simulink model "simplified_sim_2018"  (R2018b)
settings: Solver=VariableStepAuto  StartTime=0.0  StopTime=10.0  RelTol=1e-3
undefined symbols (not defined in the file or in its folder): sensors
libraries: dspindex x4, Environment_lib x1, Sensors_Lib x1, MEKF_lib x1, satelliteDynamics_lib x1
settings Model: Creator=satcave1  LastModifiedBy=kylle

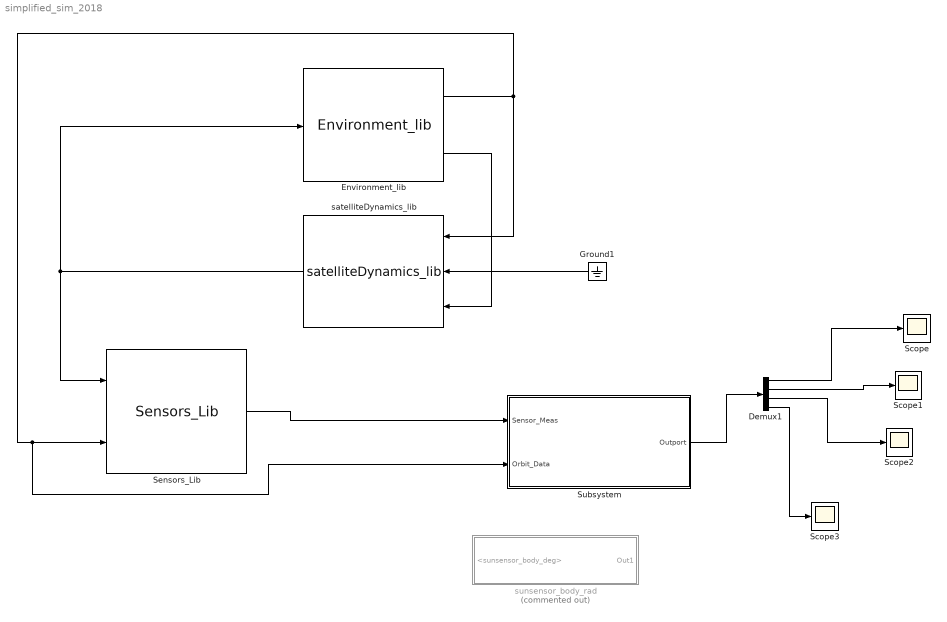
== system simplified_sim_2018 ==
  Demux1 : Demux
  Environment_lib : Environment_lib/Environment_lib  SystemSampleTime=-1
  Ground1 : Ground
  Scope{,1..3} (4 alike) : Scope
  Sensors_Lib : Sensors_Lib/Sensors_Lib  SystemSampleTime=-1
  Subsystem : Subsystem
  satelliteDynamics_lib : satelliteDynamics_lib/satelliteDynamics_lib  SystemSampleTime=-1
  sunsensor_body_rad : Subsystem  Commented=on
  wires:
  satelliteDynamics_lib/1 -> Environment_lib/1, Sensors_Lib/1
  Ground1/1 -> satelliteDynamics_lib/2
  Environment_lib/2 -> satelliteDynamics_lib/3
  Environment_lib/1 -> Subsystem/2(Orbit_Data), Sensors_Lib/2, satelliteDynamics_lib/1
  Sensors_Lib/1 -> Subsystem/1(Sensor_Meas)
  Subsystem/1(Outport) -> Demux1/1
  Demux1/1 -> Scope/1
  Demux1/2 -> Scope1/1
  Demux1/3 -> Scope2/1
  Demux1/4 -> Scope3/1

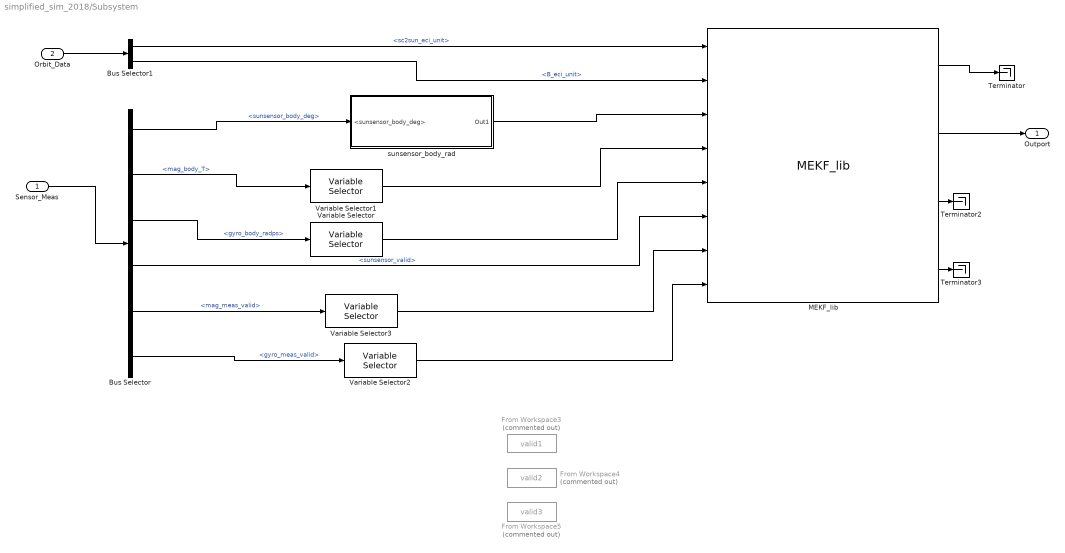
== system simplified_sim_2018/Subsystem ==
  Sensor_Meas : Inport
  Orbit_Data : Inport  Port=2
  Bus Selector : BusSelector  OutputSignals=sunsensor_body_deg,mag_body_T,gyro_body_radps,sunsensor_valid,mag_meas_valid,gyro_meas_valid
  Bus Selector1 : BusSelector  OutputSignals=sc2sun_eci_unit,B_eci_unit
  From Workspace3 : FromWorkspace  Commented=on  VariableName=valid1  SampleTime=sensors.sample_time_s
  From Workspace4 : FromWorkspace  Commented=on  VariableName=valid2  SampleTime=sensors.sample_time_s
  From Workspace5 : FromWorkspace  Commented=on  VariableName=valid3  SampleTime=sensors.sample_time_s
  MEKF_lib : MEKF_lib/MEKF_lib  SystemSampleTime=-1
  Terminator : Terminator
  Terminator2 : Terminator
  Terminator3 : Terminator
  Variable Selector : dspindex/Variable Selector  NumInputs=1  rowsOrCols=Columns  IdxMode=Fixed  Elements=[1]  ZerOneIdxMode=One-based  errmode=Clip Index  FillMode=off  FillValues=0
  Variable Selector1 : dspindex/Variable Selector  NumInputs=1  rowsOrCols=Columns  IdxMode=Fixed  Elements=[1]  ZerOneIdxMode=One-based  errmode=Clip Index  FillMode=off  FillValues=0
  Variable Selector2 : dspindex/Variable Selector  NumInputs=1  rowsOrCols=Rows  IdxMode=Fixed  Elements=[1]  ZerOneIdxMode=One-based  errmode=Clip Index  FillMode=off  FillValues=0
  Variable Selector3 : dspindex/Variable Selector  NumInputs=1  rowsOrCols=Rows  IdxMode=Fixed  Elements=[1]  ZerOneIdxMode=One-based  errmode=Clip Index  FillMode=off  FillValues=0
  sunsensor_body_rad : Subsystem
  Outport : Outport
  wires:
  MEKF_lib/1 -> Terminator/1
  MEKF_lib/2 -> Outport/1
  MEKF_lib/3 -> Terminator2/1
  MEKF_lib/4 -> Terminator3/1
  Sensor_Meas/1 -> Bus Selector/1
  Orbit_Data/1 -> Bus Selector1/1
  Bus Selector1/1 -> MEKF_lib/1  "<sc2sun_eci_unit>"
  Bus Selector1/2 -> MEKF_lib/2  "<B_eci_unit>"
  sunsensor_body_rad/1(Out1) -> MEKF_lib/3
  Bus Selector/1 -> sunsensor_body_rad/1(<sunsensor_body_deg>)  "<sunsensor_body_deg>"
  Bus Selector/3 -> Variable Selector/1  "<gyro_body_radps>"
  Bus Selector/2 -> Variable Selector1/1  "<mag_body_T>"
  Variable Selector1/1 -> MEKF_lib/4
  Variable Selector/1 -> MEKF_lib/5
  Bus Selector/4 -> MEKF_lib/6  "<sunsensor_valid>"
  Bus Selector/6 -> Variable Selector2/1  "<gyro_meas_valid>"
  Variable Selector2/1 -> MEKF_lib/8
  Bus Selector/5 -> Variable Selector3/1  "<mag_meas_valid>"
  Variable Selector3/1 -> MEKF_lib/7

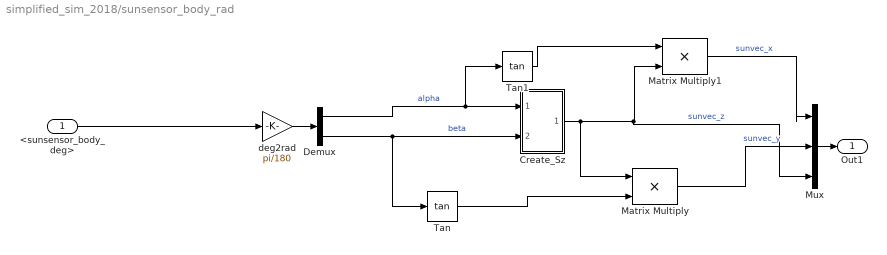
== system simplified_sim_2018/sunsensor_body_rad ==
  <sunsensor_body_deg> : Inport
  Create_Sz : Subsystem
  Demux : Demux  Outputs=2
  Matrix Multiply : Product
  Matrix Multiply1 : Product
  Mux : Mux  Inputs=3
  Tan : Trigonometry  Operator=tan
  Tan1 : Trigonometry  Operator=tan
  deg2rad : Gain  Gain=pi/180
  Out1 : Outport
  wires:
  Tan/1 -> Matrix Multiply/2
  Demux/1 -> Tan1/1, Create_Sz/1(alpha)  "alpha"
  Matrix Multiply/1 -> Mux/2  "sunvec_y"
  Create_Sz/1(Out1) -> Mux/3, Matrix Multiply1/2, Matrix Multiply/1  "sunvec_z"
  Demux/2 -> Tan/1, Create_Sz/2(beta)  "beta"
  Tan1/1 -> Matrix Multiply1/1
  deg2rad/1 -> Demux/1
  Mux/1 -> Out1/1
  Matrix Multiply1/1 -> Mux/1  "sunvec_x"
  <sunsensor_body_deg>/1 -> deg2rad/1

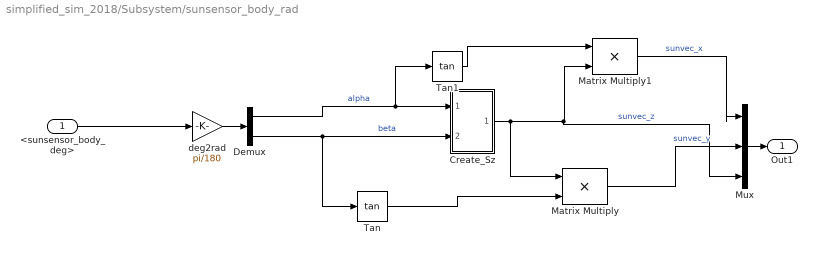
== system simplified_sim_2018/Subsystem/sunsensor_body_rad ==
  <sunsensor_body_deg> : Inport
  Create_Sz : Subsystem
  Demux : Demux  Outputs=2
  Matrix Multiply : Product
  Matrix Multiply1 : Product
  Mux : Mux  Inputs=3
  Tan : Trigonometry  Operator=tan
  Tan1 : Trigonometry  Operator=tan
  deg2rad : Gain  Gain=pi/180
  Out1 : Outport
  wires:
  Tan/1 -> Matrix Multiply/2
  Demux/1 -> Tan1/1, Create_Sz/1(alpha)  "alpha"
  Matrix Multiply/1 -> Mux/2  "sunvec_y"
  Create_Sz/1(Out1) -> Mux/3, Matrix Multiply1/2, Matrix Multiply/1  "sunvec_z"
  Demux/2 -> Tan/1, Create_Sz/2(beta)  "beta"
  Tan1/1 -> Matrix Multiply1/1
  deg2rad/1 -> Demux/1
  Mux/1 -> Out1/1
  Matrix Multiply1/1 -> Mux/1  "sunvec_x"
  <sunsensor_body_deg>/1 -> deg2rad/1

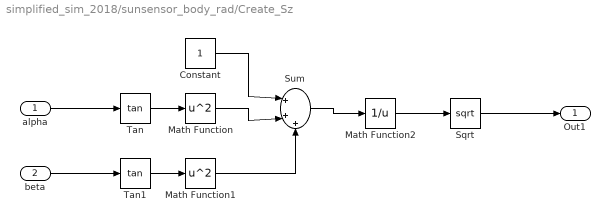
== system simplified_sim_2018/sunsensor_body_rad/Create_Sz ==
  alpha : Inport
  beta : Inport  Port=2
  Constant : Constant
  Math Function : Math  Operator=square  SaturateOnIntegerOverflow=on
  Math Function1 : Math  Operator=square  SaturateOnIntegerOverflow=on
  Math Function2 : Math  Operator=reciprocal  SaturateOnIntegerOverflow=on
  Sqrt : Sqrt  SaturateOnIntegerOverflow=on
  Sum : Sum  Inputs=|+++
  Tan : Trigonometry  Operator=tan
  Tan1 : Trigonometry  Operator=tan
  Out1 : Outport
  wires:
  Constant/1 -> Sum/1
  Sum/1 -> Math Function2/1
  Tan/1 -> Math Function/1
  Math Function/1 -> Sum/2
  Math Function2/1 -> Sqrt/1
  Tan1/1 -> Math Function1/1
  alpha/1 -> Tan/1
  beta/1 -> Tan1/1
  Math Function1/1 -> Sum/3
  Sqrt/1 -> Out1/1

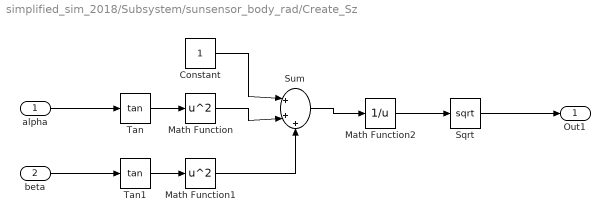
== system simplified_sim_2018/Subsystem/sunsensor_body_rad/Create_Sz ==
  alpha : Inport
  beta : Inport  Port=2
  Constant : Constant
  Math Function : Math  Operator=square  SaturateOnIntegerOverflow=on
  Math Function1 : Math  Operator=square  SaturateOnIntegerOverflow=on
  Math Function2 : Math  Operator=reciprocal  SaturateOnIntegerOverflow=on
  Sqrt : Sqrt  SaturateOnIntegerOverflow=on
  Sum : Sum  Inputs=|+++
  Tan : Trigonometry  Operator=tan
  Tan1 : Trigonometry  Operator=tan
  Out1 : Outport
  wires:
  Constant/1 -> Sum/1
  Sum/1 -> Math Function2/1
  Tan/1 -> Math Function/1
  Math Function/1 -> Sum/2
  Math Function2/1 -> Sqrt/1
  Tan1/1 -> Math Function1/1
  alpha/1 -> Tan/1
  beta/1 -> Tan1/1
  Math Function1/1 -> Sum/3
  Sqrt/1 -> Out1/1
